simulink model "osqp_mpccontroller_example"  (R2018a)
settings: Solver=VariableStepAuto  StartTime=0.0  StopTime=10.0  RelTol=1e-3
values from neighbouring files (symbols this model uses):
  Ad = [1       0       0   0   0   0   0.1     0       0    0       0       0 ... (first row only)    [osqp_mpccontroller.m]    (also in plant.m)
  Bd = [0      -0.0726  0       0.0726 ... (first row only)    [osqp_mpccontroller.m]    (also in plant.m)
settings Model: Creator=gluo  LastModifiedBy=gluo

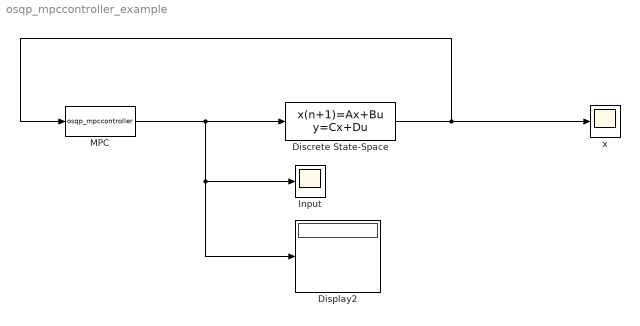
== system osqp_mpccontroller_example ==
  Discrete State-Space : DiscreteStateSpace  A=Ad  B=Bd  C=eye(length(Ad))  D=zeros(size(Bd))  InitialCondition=zeros(12,1)  SampleTime=0.01
  Display2 : Display
  Input : Scope
  MPC : MATLABFcn  MATLABFcn=osqp_mpccontroller  OutputDimensions=4  Output1D=off
  x : Scope
  wires:
  Discrete State-Space/1 -> x/1, MPC/1
  MPC/1 -> Discrete State-Space/1, Input/1, Display2/1
